simulink model "nivel_1"  (R2023b)
settings: Solver=FixedStepAuto  StartTime=0.0  StopTime=60  FixedStep=0.001  RelTol=1e-3
undefined symbols (not defined in the file): b_cx, b_cy, b_hb, b_hEb, b_hwu, b_t, b_tb, b_tw, bh_eq, bh_eq_prima, bt_eq, CI, ddx_t_lim, ddy_h_lim, DiscIntNeverNeededParam, dx_t_lim, dy_h_lim, g, H_c, H_SS, i_h, i_t, Jh_eq, Jh_eq_aux, Jt_eq, K_cy, K_hwu, K_tw, Kd_h, Kd_t, Ki_h, Ki_t, Kp_h, Kp_t, L_h0, M_cmax, M_s, m_t, r_hd, r_td, T_hb_max, T_hEb_max, T_hm_max, T_s1, T_s2, T_tb_max, T_tm_max, tau_hm, tau_tm, W_c, x_t_lim, Y_c, y_h_lim, Y_t0
libraries: simulink x19, dspstat3 x1, sldrtlib x1, simulink_extras x1
(part 2 of 2)

== stateflow chart nivel_1/Nivel 1 ==
  state Controlador
    entry:
    y_c = Y_c;
    state Mapeo_entradas_digitales [parallel]
      during:
      % Seleccion de operacion
      seleccion_oper = inputs(1);
      % Seleccion de muelle
      n_muelle = inputs(2);
      % Seleccion de posiciones en barco (+1 por sill beam)
      p_ini = inputs(3) + 1;
      p_fin = inputs(4) + 1;
      % Comandos del joystick
      joy_up = inputs(5);
      joy_down = inputs(6);
      % Modo de twistlocks (TLK)
      modo_tlk = inputs(7);
      % Inicio de operacion
      ini_oper = inputs(8);
      % Limit switches
      LLS_xt = limit_switches(1);
      RLS_xt = limit_switches(2);
      LELS_xt = limit_switches(3);
      RELS_xt = limit_switches(4);
      LLS_yt = limit_switches(5);
      RLS_yt = limit_switches(6);
      LELS_yt = limit_switches(7);
      RELS_yt = limit_switches(8);
      OS_izaje = limit_switches(15);
      settings: executionOrder=1
    state Operacion [parallel]
      settings: executionOrder=2
      note: Segun seleccion del operario
          | 0. Volver a home
          | Buscar carga en el muelle y llevar al barco
          | Buscar carga en barco y llevar al muelle
          | Mover carga dentro del barco
          | Reconocimiento de obstaculos
      state StandBy_home
        % Spreader en posicion de home
        % Espera hasta que el operador seleccione una operacion y la inicie
        % Siempre frenos puestos
        entry:
        BRK_h = false;
        BRK_t = false;
        fin_oper = false;
      state Reconocimiento_obstaculos
        % Se realiza recorrido desde x = 0 hasta limite (x = 50 - W_c/2) y se vuelve a posicion de SB (x = 0)
        entry:
        [x_t_vec, dx_t_vec] = perfil_velocidad_trapezoidal(T_s1, 0, 0, (x_t_lim(2) - W_c/2) ,0, set_param_lim(3), set_param_lim(4));
        BRK_t = true;
        flag_recon = 0;
        state Recorrido
          entry:
          idx_t = 1;
          during:
          % Paso de consigna de CARRO
          x_t = x_t_vec(idx_t);
          dx_t = dx_t_vec(idx_t);
          if idx_t  ~=  length(x_t_vec)
          idx_t = idx_t + 1;
          else
          flag_recon = flag_recon + 1;
          end
        state Vuelta
          entry:
          x_t_vec = flip(x_t_vec);
          dx_t_vec = -dx_t_vec;
          flag_recon = flag_recon + 1;
        (default) -> Recorrido
        Recorrido -> Vuelta : [flag_recon == 1]
        Vuelta -> Recorrido
      state Posicionamiento_desde_home
        % Se posiciona el spreader segun el tipo de accion partiendo desde home
        % Segun la seleccion del oeprador hay que posicionarse en muelle o barco
        % En funciones de homing, TIPO
        %     0 ->  IR A HOME
        %     1 -> SALIR DESDE HOME
        state StandBy
          entry:
          % Se abren frenos de izaje y carro
          BRK_h = true;
          BRK_t = true;
          flag = 0;
        state A_muelle
          entry:
          [carro_cons, izaje_cons, t_brk_t] = homing_muelle(T_s1, y_c_alt, W_c, H_c, set_param_lim, H_SS, tipo, n_muelle, -set_param_lim(3) * 0.5);
        state Salida_consignas
          entry:
          idx = 1;
          flag = 0;
          t_aux = clock;
          % =======================
          during:
          % Consignas de carro
          x_t = carro_cons(idx, 1);
          dx_t = carro_cons(idx, 2);
          % Consignas de izaje
          y_h = izaje_cons(idx, 1);
          dy_h = izaje_cons(idx, 2);
          if idx  ~=  length(izaje_cons)
          idx = idx + 1;
          end
          if idx == length(carro_cons)
          flag = 1;
          end
          % Freno de carro en caso de ser necesario
          if clock - t_aux > t_brk_t
          BRK_t = false;
          end
        state A_barco
          entry:
          [carro_cons, izaje_cons, t_brk_t] = homing_barco(T_s1, y_c_alt, W_c, set_param_lim, 1.5 * H_SS, tipo, p_ini, -1);
        (default) -> Controlador.Operacion.Posicionamiento_desde_home.StandBy
        Controlador.Operacion.Posicionamiento_desde_home.StandBy -> Controlador.Operacion.Posicionamiento_desde_home.A_muelle [order 2] : [seleccion_oper == 1]
        Controlador.Operacion.Posicionamiento_desde_home.A_muelle -> Controlador.Operacion.Posicionamiento_desde_home.Salida_consignas
        Controlador.Operacion.Posicionamiento_desde_home.StandBy -> Controlador.Operacion.Posicionamiento_desde_home.A_barco [order 1] : [seleccion_oper == 2]
        Controlador.Operacion.Posicionamiento_desde_home.A_barco -> Controlador.Operacion.Posicionamiento_desde_home.Salida_consignas
      state Posicionamiento_a_homing
        % Se posiciona el spreader segun el tipo de accion partiendo desde home
        % Segun la seleccion del oeprador hay que posicionarse en muelle o barco
        % En funciones de homing, TIPO
        %     0 ->  IR A HOME
        %     1 -> SALIR DESDE HOME
        tipo = 1;
        state StandBy
          entry:
          % Se abren frenos de izaje y carro
          BRK_h = true;
          BRK_t = true;
          flag = 0;
        state A_muelle
          entry:
          [carro_cons, izaje_cons, t_brk_t] = homing_muelle(T_s1, y_c_alt, W_c, H_c, set_param_lim, H_SS, tipo, n_muelle, -set_param_lim(3) * 0.5);
        state Salida_consignas
          entry:
          idx = 1;
          flag = 0;
          t_aux = clock;
          % =======================
          during:
          % Consignas de carro
          x_t = carro_cons(idx, 1);
          dx_t = carro_cons(idx, 2);
          % Consignas de izaje
          y_h = izaje_cons(idx, 1);
          dy_h = izaje_cons(idx, 2);
          if idx  ~=  length(izaje_cons)
          idx = idx + 1;
          end
          if idx == length(carro_cons)
          flag = 1;
          end
          % Freno de carro en caso de ser necesario
          if clock - t_aux > t_brk_t
          BRK_t = false;
          end
        state A_barco
          entry:
          [carro_cons, izaje_cons, t_brk_t] = homing_barco(T_s1, y_c_alt, W_c, set_param_lim, 1.5 * H_SS, tipo, p_ini, -1);
        (default) -> Controlador.Operacion.Posicionamiento_a_homing.StandBy
        Controlador.Operacion.Posicionamiento_a_homing.StandBy -> Controlador.Operacion.Posicionamiento_a_homing.A_muelle [order 2] : [seleccion_oper == 1]
        Controlador.Operacion.Posicionamiento_a_homing.A_muelle -> Controlador.Operacion.Posicionamiento_a_homing.Salida_consignas
        Controlador.Operacion.Posicionamiento_a_homing.StandBy -> Controlador.Operacion.Posicionamiento_a_homing.A_barco [order 1] : [seleccion_oper == 2]
        Controlador.Operacion.Posicionamiento_a_homing.A_barco -> Controlador.Operacion.Posicionamiento_a_homing.Salida_consignas
      note: Los pasos en las operaciones (una vez se realizo el posicionamiento) se enumeran como
          | Descenso manual
          | Cambio en modo de TLK (cierre)
          | Ascenso manual
          | Operacion automatica
          | Vuelta al paso 1
      state Modo_manual
        state Comprobacion_carga
          % Se realiza una comprobacion del peso del container al momento de realizar el izaje
          entry:
          t_aux = clock;
          state Levantamiento_carga
            % Se acelera hasta llegar a velocidad constante y se comprueba el peso
            during:
            if dy_h <= 0.5
            dy_h = (ddy_h_lim_man * T_s1) + dy_h;
            end
            y_h = p_izaje - H_c;
          state Descenso_por_sobrecarga
            % Se realiza descenso en velocidad reducida hasta F_hw = 0
            % y se activa alarma por sobrecarga
            during:
            if dy_h >= -0.5
            dy_h = -(ddy_h_lim * T_s1) + dy_h;
            end
            y_h = p_izaje - H_c;
            sobrecarga = true;
          state Calculo_carga
            % Calculo de tolerancia maxima de 5%
            entry:
            tol = M_cmax * 0.05;
            M_calc = (((2* F_hw) / g) - M_s);
          (default) -> Controlador.Operacion.Modo_manual.Comprobacion_carga.Levantamiento_carga
          Controlador.Operacion.Modo_manual.Comprobacion_carga.Levantamiento_carga -> Controlador.Operacion.Modo_manual.Comprobacion_carga.Calculo_carga : [clock - t_aux >= 3]
          Controlador.Operacion.Modo_manual.Comprobacion_carga.Calculo_carga -> Descenso_por_sobrecarga [order 1] : [M_calc >= M_cmax + tol]
        state StandBy
          % Se espera comando de subida o de bajada
          % Existen dos casos dentro del modo manual
          %    1 - Descenso desde altura segura, se limita seguridad
          %         Se realiza paro por inactividad del operario
          %         El descenso manual finaliza cuando F_hw == 0 (apoyo)
          %    2 - Ascenso hasta altura segura, se limita la velocidad de izaje
          % ==============
          entry:
          % Limites en la aceleracion y velocidad de izaje
          dy_h_lim_man = set_param_lim(3) * 0.5;
          ddy_h_lim_man = set_param_lim(4) * 0.5;
          y_h_aux = p_izaje;
        state Paro_inactividad
          % En caso de no tomar los controles se desacelera y se frena en v_0
          during:
          if dy_h <= 0
          dy_h = (ddy_h_lim_man * T_s1) + dy_h;
          else
          dy_h = 0;
          BRK_h = false;
          end
          y_h = p_izaje - (TLK * H_c);
        state Descenso_manual
          % Se realiza descenso progresivo hasta que se haga contacto con el container (F_hw == 0)
          % El descenso es a velocidad limitada, por cada que se mueve la palanca se genera una rampa de velocidad
          state Rampa_desc_velocidad
            during:
            dy_h = -(ddy_h_lim_man * T_s1) + dy_h;
            y_h = p_izaje - (TLK * H_c);
          state Rampa_asc_velocidad
            during:
            dy_h = (ddy_h_lim_man * T_s1) + dy_h;
            y_h = p_izaje - (TLK * H_c);
          state V_ctte
            during:
            y_h = p_izaje - (TLK * H_c);
            if dy_h >= 0
            dy_h = 0;
            elseif dy_h <= -dy_h_lim_man
            dy_h = -dy_h_lim_man;
            end
          (default) -> Controlador.Operacion.Modo_manual.Descenso_manual.Rampa_desc_velocidad
          Controlador.Operacion.Modo_manual.Descenso_manual.Rampa_desc_velocidad -> Controlador.Operacion.Modo_manual.Descenso_manual.Rampa_asc_velocidad [order 1] : [joy_down == 0]
          Controlador.Operacion.Modo_manual.Descenso_manual.Rampa_asc_velocidad -> Controlador.Operacion.Modo_manual.Descenso_manual.Rampa_desc_velocidad [order 2] : [joy_down == 1 && dy_h > -dy_h_lim_man]
          Controlador.Operacion.Modo_manual.Descenso_manual.V_ctte -> Controlador.Operacion.Modo_manual.Descenso_manual.Rampa_desc_velocidad [order 2] : [joy_down == 1 && dy_h < -dy_h_lim_man]
          Controlador.Operacion.Modo_manual.Descenso_manual.Rampa_desc_velocidad -> Controlador.Operacion.Modo_manual.Descenso_manual.V_ctte [order 2] : [dy_h <= -dy_h_lim_man]
          Controlador.Operacion.Modo_manual.Descenso_manual.Rampa_asc_velocidad -> Controlador.Operacion.Modo_manual.Descenso_manual.V_ctte [order 1] : [dy_h >= 0]
          Controlador.Operacion.Modo_manual.Descenso_manual.V_ctte -> Controlador.Operacion.Modo_manual.Descenso_manual.Rampa_asc_velocidad [order 1] : [joy_down == 0 && dy_h ~= 0]
        state Ascenso_manual
          % Se realiza descenso progresivo hasta que se haya contacto con el container (F_hw == 0)
          % El descenso es a velocidad limitada, por cada que se mueve la palanca se genera una rampa de velocidad
          paso = 3;
          state Rampa_asc_velocidad
            during:
            dy_h = (ddy_h_lim_man * T_s1) + dy_h;
            y_h = p_izaje - (TLK * H_c);
          state Rampa_desc_velocidad
            during:
            dy_h = -(ddy_h_lim_man * T_s1) + dy_h;
            y_h = p_izaje - (TLK * H_c);
          state V_ctte
            during:
            y_h = p_izaje - (TLK * H_c);
            if dy_h <= 0
            dy_h = 0;
            elseif dy_h >= dy_h_lim_man
            dy_h = dy_h_lim_man;
            end
          (default) -> Controlador.Operacion.Modo_manual.Ascenso_manual.Rampa_asc_velocidad
          Controlador.Operacion.Modo_manual.Ascenso_manual.Rampa_asc_velocidad -> Controlador.Operacion.Modo_manual.Ascenso_manual.Rampa_desc_velocidad [order 2] : [joy_up == 0]
          Controlador.Operacion.Modo_manual.Ascenso_manual.Rampa_desc_velocidad -> Controlador.Operacion.Modo_manual.Ascenso_manual.Rampa_asc_velocidad [order 2] : [joy_up == 1 && dy_h < dy_h_lim_man]
          Controlador.Operacion.Modo_manual.Ascenso_manual.V_ctte -> Controlador.Operacion.Modo_manual.Ascenso_manual.Rampa_asc_velocidad [order 2] : [joy_up == 1 && dy_h < dy_h_lim_man]
          Controlador.Operacion.Modo_manual.Ascenso_manual.Rampa_asc_velocidad -> Controlador.Operacion.Modo_manual.Ascenso_manual.V_ctte [order 1] : [dy_h >= dy_h_lim_man]
          Controlador.Operacion.Modo_manual.Ascenso_manual.Rampa_desc_velocidad -> Controlador.Operacion.Modo_manual.Ascenso_manual.V_ctte [order 1] : [dy_h <= 0]
          Controlador.Operacion.Modo_manual.Ascenso_manual.V_ctte -> Controlador.Operacion.Modo_manual.Ascenso_manual.Rampa_desc_velocidad [order 1] : [joy_up == 0 && dy_h ~= 0]
        (default) -> Controlador.Operacion.Modo_manual.StandBy
        (junction 383) -> Controlador.Operacion.Modo_manual.Comprobacion_carga [order 1] : [TLK == true]
        Controlador.Operacion.Modo_manual.StandBy -> (junction 383) [order 1] : [joy_up == 1 && paso == 2]
            | {BRK_h = true,
            | paso = 3;}
        (junction 383) -> Controlador.Operacion.Modo_manual.Ascenso_manual [order 2] : [TLK == false ]
        Controlador.Operacion.Modo_manual.Comprobacion_carga.Calculo_carga -> Controlador.Operacion.Modo_manual.Ascenso_manual [order 2] : [M_calc < M_cmax + tol]
        Controlador.Operacion.Modo_manual.StandBy -> (junction 327) [order 2] : [paso == 1]
        (junction 327) -> Controlador.Operacion.Modo_manual.Paro_inactividad [order 1] : [joy_down == 0]
        (junction 327) -> Controlador.Operacion.Modo_manual.Descenso_manual [order 2] : [joy_down == 1]
        Controlador.Operacion.Modo_manual.Paro_inactividad -> Controlador.Operacion.Modo_manual.Descenso_manual : [joy_down == 1]
            | {BRK_h = true;}
      state StandBy_posicionado
        % Spreader en posicion fuera de home (muelle o barco)
        % Espera hasta que el operador seleccione una operacion y la inicie
        % Siempre frenos puestos
        entry:
        BRK_h = false;
        BRK_t = false;
        fin_oper = false;
      state Apoyo
        % Dependiendo de los TLK
        %    TLK = true -> container apoyado
        %    TLK = false -> spreader apoyado
        % Se aplica freno de izaje y se espera a comando del operador
        entry:
        fin_modo_TLK = false;
        y_h = p_izaje - (TLK * H_c);
        dy_h = 0;
        paso = 2;
        state Cierre_TLK
          % Se pretende tomar una carga
          % Se simula el cierre con 3 segundos de delay
          entry:
          t_aux = clock;
          exit:
          TLK = true;
          if seleccion_oper == 2
          y_c(pos_x) = y_c(pos_x) - 1;
          end
        state StandBy
          % A la espera del comando del operador
        state Fin_modo_TLK
          fin_modo_TLK = true;
        state Apertura_TLK
          % Se pretende soltar la carga
          % Se simula la apertura con 3 segundos de delay
          entry:
          t_aux = clock;
          exit:
          TLK = false;
          y_c(p_ini) = y_c(p_ini) + 1;
          fin_oper = true;
          if seleccion_oper == 1
          y_c(pos_x) = y_c(pos_x) + 1;
          end
        Controlador.Operacion.Apoyo.StandBy -> Controlador.Operacion.Apoyo.Cierre_TLK [order 2] : [TLK == false && modo_tlk == 1]
        (default) -> Controlador.Operacion.Apoyo.StandBy
        Controlador.Operacion.Apoyo.Cierre_TLK -> Controlador.Operacion.Apoyo.Fin_modo_TLK : [(clock - t_aux) >= 3 ]
        Controlador.Operacion.Apoyo.StandBy -> Controlador.Operacion.Apoyo.Apertura_TLK [order 1] : [TLK == true && modo_tlk == 0]
        Controlador.Operacion.Apoyo.Apertura_TLK -> Controlador.Operacion.Apoyo.Fin_modo_TLK : [(clock - t_aux) >= 3]
      state Modo_automatico
        % Dependiendo del tipo de operacion (seleccion_oper) se cambia el valor del tipo
        %     tipo = 0 -> Descarga desde barco al muelle
        %     tipo = 1 -> Carga desde muelle a barco
        %     tipo = 2 -> Movimiento dentro del barco
        % Luego se utiliza la variable paso para determinar si es posicionamiento o toma de carga/descarga
        state Salida_consignas
          entry:
          idx = 1;
          flag = 0;
          t_aux = clock;
          % =======================
          during:
          % Consignas de carro
          x_t = carro_cons(idx, 1);
          dx_t = carro_cons(idx, 2);
          % Consignas de izaje
          y_h = izaje_cons(idx, 1);
          dy_h = izaje_cons(idx, 2);
          if idx  ~=  length(izaje_cons)
          idx = idx + 1;
          end
          if idx == length(carro_cons)
          flag = 1;
          end
          % Freno de carro en caso de ser necesario
          if clock - t_aux > t_brk_t
          BRK_t = false;
          end
        state Condicionantes
          entry:
          if seleccion_oper == 0
          % Descarga desde barco a muelle
          tipo = 0;
          elseif seleccion_oper == 1
          % Carga desde muelle a barco
          tipo = 1;
          else
          % Operacion intra-barco
          tipo = 2;
          end
        state Consignas_automatico
          entry:
          [carro_cons, izaje_cons, t_brk_t, t_brk_h] = operacion_automatico(T_s1, y_c_alt, W_c, H_c, TLK, set_param_lim, H_SS, tipo, n_muelle, p_ini, p_fin, dy_h, set_param_lim(3));
        (default) -> Controlador.Operacion.Modo_automatico.Condicionantes
        Controlador.Operacion.Modo_automatico.Condicionantes -> Consignas_automatico
        Consignas_automatico -> Controlador.Operacion.Modo_automatico.Salida_consignas
      state Posicionamiento_automatico
        % El spreader esta fuera de homing, pero o esta dentro del barco o en muelle
        % Entonces dependiende de la seleccion del operador, y las condiciones de posicionamiento del spreader, se usa una de las siguientes funciones
        %
        % Spreader esta en barco y operador selecciona operacion de muelle a barco (o viceversa, spreader en muelle y operacion barco a muelle)
        %   operacion_automatico (tipo 0 y 1)
        %
        % Spreader esta en barco y operador selecciona de barco a muelle
        %   operacion_automatico (tipo 2)
        %
        % Spreader esta en muelle y operador selecciona de muelle a barco
        %   cambia_muelle
        entry:
        BRK_t = true;
        BRK_h = true;
        state Salida_consignas
          entry:
          idx = 1;
          flag = 0;
          t_aux = clock;
          % =======================
          during:
          % Consignas de carro
          x_t = carro_cons(idx, 1);
          dx_t = carro_cons(idx, 2);
          % Consignas de izaje
          y_h = izaje_cons(idx, 1);
          dy_h = izaje_cons(idx, 2);
          if idx  ~=  length(izaje_cons)
          idx = idx + 1;
          end
          if idx == length(carro_cons)
          flag = 1;
          end
          % Freno de carro en caso de ser necesario
          if clock - t_aux > t_brk_t
          BRK_t = false;
          end
        state Condicionantes
          entry:
          tipo = -1;
          if x_t < 0 && seleccion_oper == 2 || seleccion_oper == 3
          tipo = 1;
          elseif x_t > 0 && seleccion_oper == 1
          tipo = 0;
          elseif x_t > 0 && seleccion_oper == 3
          tipo = 2;
          end
        state Posicionamiento_en_muelle
          entry:
          % Calculo del muelle actual
          n_muelle_act = fix(abs(p_carro) / (2 * W_c)) + 1;
          [carro_cons, izaje_cons, t_brk_t, t_brk_h] = cambio_muelle(T_s1, W_c, H_c, set_param_lim, H_SS, n_muelle_act, n_muelle, 0)
        state Posicionamiento_combinado
          entry:
          [carro_cons, izaje_cons, t_brk_t, t_brk_h] = operacion_automatico(T_s1, y_c_alt, W_c, H_c, TLK, set_param_lim, H_SS, tipo, n_muelle, p_ini, p_fin, dy_h, set_param_lim(3));
        Posicionamiento_en_muelle -> Controlador.Operacion.Posicionamiento_automatico.Salida_consignas
        (default) -> Controlador.Operacion.Posicionamiento_automatico.Condicionantes
        Controlador.Operacion.Posicionamiento_automatico.Condicionantes -> Posicionamiento_en_muelle [order 1] : [tipo == -1]
        Posicionamiento_combinado -> Controlador.Operacion.Posicionamiento_automatico.Salida_consignas
        Controlador.Operacion.Posicionamiento_automatico.Condicionantes -> Posicionamiento_combinado [order 2] : [tipo ~= -1]
      (default) -> StandBy_home
      StandBy_home -> Reconocimiento_obstaculos [order 2] : [seleccion_oper == 4 && ini_oper == 1]
      Posicionamiento_a_homing -> StandBy_home : [flag == 1]
      Reconocimiento_obstaculos -> StandBy_home : [flag_recon == 3]
          | {flag_recon = 0;}
      StandBy_home -> Posicionamiento_desde_home [order 1] : [(seleccion_oper >= 1 && seleccion_oper <= 3) && ini_oper == 1]
      StandBy_posicionado -> Posicionamiento_a_homing [order 1] : [seleccion_oper == 0 && ini_oper == 1]
      Posicionamiento_desde_home -> Controlador.Operacion.Modo_manual : [flag == 1]
          | {paso = 1;}
      Controlador.Operacion.Modo_manual -> Apoyo [order 1] : [F_hw == 0]
          | {BRK_h = false;}
      Controlador.Operacion.Modo_manual -> StandBy_posicionado [order 3] : [((y_h_aux + H_SS) <= (y_h + (TLK * H_c))) && fin_oper == true]
      Apoyo -> Controlador.Operacion.Modo_manual : [fin_modo_TLK == true]
      Posicionamiento_automatico -> Controlador.Operacion.Modo_manual : [flag == 1]
          | {paso = 1;}
      StandBy_posicionado -> Posicionamiento_automatico [order 2] : [(seleccion_oper >= 1 && seleccion_oper <= 3) && ini_oper == 1]
      Controlador.Operacion.Modo_automatico -> Controlador.Operacion.Modo_manual : [flag == 1]
          | {paso = 1;}
      Controlador.Operacion.Modo_manual -> Controlador.Operacion.Modo_automatico [order 2] : [paso == 3 && ((y_h_aux + H_SS) <= (y_h + (TLK * H_c))) ]
          | {BRK_t = true;
          | paso = 4;}
    state Mapeo_entradas_analogicas [parallel]
      during:
      % Sensores en motores
      p_carro = sensores(1);
      v_carro = sensores(2);
      p_izaje = sensores(3);
      v_izaje = sensores(4);
      settings: executionOrder=3
    state Mapeo_salidas_analogicas [parallel]
      during:
      % Calculo de y_c0 -------------------------
      pos_x = fix(abs(x_t / (2 * W_c))) + 1;
      % Encima de barco
      if x_t > 0 && pos_x <= length(y_c)
      y_c0 = y_c_alt(pos_x);
      % Fuera del barco
      elseif x_t < 0
      y_c0 = H_c * (~TLK);
      end
      % Calculo del peso de la carga
      M_calc_aux = ((2* F_hw) / g) - M_s;
      if M_calc_aux > M_cmax
      M_calc_aux = M_cmax;
      end
      settings: executionOrder=4
    state Auxiliares [parallel]
      during:
      % Segun modo de twistlocks se calculan limites de velocidad de izaje
      if TLK == true
      h_c = H_c;
      % Interpolacion para velocidad maxima segun la carga
      v_lim_carga = dy_h_lim(1) + (dy_h_lim(2) - dy_h_lim(1)) * (M_calc_aux / M_cmax);
      set_param_lim = [dx_t_lim ddx_t_lim v_lim_carga ddy_h_lim];
      else
      h_c = 0;
      set_param_lim = [dx_t_lim ddx_t_lim dy_h_lim(2) ddy_h_lim];
      end
      % Perfil de obstaculos en [m]
      y_c_alt = y_c * H_c;
      settings: executionOrder=5
  state Modo_manual [commented out]
    % En este estado se comanda la logica en modo manual, solo en casos de carga y descarga de containers
    state StandBy [commented out]
      % Existen tres casos dentro del modo manual
      %    1 - Descenso (v_h < 0)
      %    2 - Ascenso (cuando se carga/descarga)
      %    3 - Toma de carga (manejo de TLK)
    state Paro_inactividad [commented out]
      % En caso de no tomar los controles se aplican frenos y se espera comando del operador
      during:
      if dy_h < 0
      dy_h = (ddy_h_lim * T_s1) + dy_h;
      else
      dy_h = 0;
      BRK_h = false;
      end
      y_h = p_izaje;
    state Descenso_manual [commented out]
      % Se realiza descenso progresivo hasta que se haya contacto con el container (F_hw == 0)
      % El descenso es a velocidad limitada, por cada que se mueve la palanca se genera una rampa de velocidad
      entry:
      v_limite = -dy_h_lim(1);
      state Rampa_asc_velocidad [commented out]
        during:
        dy_h = -(ddy_h_lim * T_s1) + dy_h;
        y_h = p_izaje - (TLK * H_c);
      state Rampa_desc_velocidad [commented out]
        during:
        dy_h = (ddy_h_lim * T_s1) + dy_h;
        y_h = p_izaje - (TLK * H_c);
      state V_ctte [commented out]
        during:
        y_h = p_izaje - (TLK * H_c);
        if dy_h >= 0
        dy_h = 0;
        elseif dy_h <= v_limite
        dy_h = v_limite;
        end
      (default) -> Modo_manual.Descenso_manual.Rampa_asc_velocidad [commented out]
      Modo_manual.Descenso_manual.Rampa_asc_velocidad -> Modo_manual.Descenso_manual.Rampa_desc_velocidad [commented out] : [joy_down == 0]
      Modo_manual.Descenso_manual.Rampa_desc_velocidad -> Modo_manual.Descenso_manual.Rampa_asc_velocidad [commented out] : [joy_down == 1 && dy_h > v_limite]
      Modo_manual.Descenso_manual.V_ctte -> Modo_manual.Descenso_manual.Rampa_asc_velocidad [commented out] : [joy_down == 1 && dy_h > v_limite]
      Modo_manual.Descenso_manual.Rampa_asc_velocidad -> Modo_manual.Descenso_manual.V_ctte [commented out] : [dy_h <= v_limite]
      Modo_manual.Descenso_manual.V_ctte -> Modo_manual.Descenso_manual.Rampa_desc_velocidad [commented out] : [joy_down == 0 && dy_h ~= 0]
      Modo_manual.Descenso_manual.Rampa_desc_velocidad -> Modo_manual.Descenso_manual.V_ctte [commented out] : [dy_h >= 0]
    state Ascenso_manual [commented out]
      % Se realiza descenso progresivo hasta que se haya contacto con el container (F_hw == 0)
      % El descenso es a velocidad limitada, por cada que se mueve la palanca se genera una rampa de velocidad
      entry:
      v_limite = set_param_lim(3);
      state Rampa_asc_velocidad [commented out]
        during:
        dy_h = ddy_h_lim * T_s1 + dy_h;
        y_h = p_izaje - (TLK * H_c);
      state Rampa_desc_velocidad [commented out]
        during:
        dy_h = -(ddy_h_lim * T_s1) + dy_h;
        y_h = p_izaje - (TLK * H_c);
      state V_ctte [commented out]
        during:
        y_h = p_izaje - (TLK * H_c);
        if dy_h <= 0
        dy_h = 0;
        elseif dy_h >= v_limite
        dy_h = v_limite;
        end
      (default) -> Modo_manual.Ascenso_manual.Rampa_asc_velocidad [commented out]
      Modo_manual.Ascenso_manual.Rampa_asc_velocidad -> Modo_manual.Ascenso_manual.Rampa_desc_velocidad [commented out] : [joy_up == 0]
      Modo_manual.Ascenso_manual.Rampa_desc_velocidad -> Modo_manual.Ascenso_manual.Rampa_asc_velocidad [commented out] : [joy_up == 1 && dy_h < v_limite]
      Modo_manual.Ascenso_manual.V_ctte -> Modo_manual.Ascenso_manual.Rampa_asc_velocidad [commented out] : [joy_up == 1 && dy_h < v_limite]
      Modo_manual.Ascenso_manual.Rampa_asc_velocidad -> Modo_manual.Ascenso_manual.V_ctte [commented out] : [dy_h >= v_limite]
      Modo_manual.Ascenso_manual.V_ctte -> Modo_manual.Ascenso_manual.Rampa_desc_velocidad [commented out] : [joy_up == 0 && dy_h ~= 0]
      Modo_manual.Ascenso_manual.Rampa_desc_velocidad -> Modo_manual.Ascenso_manual.V_ctte [commented out] : [dy_h <= 0]
    state Apoyo_en_container [commented out]
      % Spreader apoyado en container, se procede a poner freno en izaje y enviar consigna de velocidad 0
      entry:
      BRK_h = false;
      y_h = p_izaje;
      dy_h = 0;
      state Cierre_TLK [commented out]
        % Se pretende tomar una carga
        % Se simula el cierre con 3 segundos de delay
        entry:
        t_aux = clock;
        exit:
        TLK = true;
      state StandBy [commented out]
        % A la espera en el
        % cambio en
        % modo_tlk
      state Fin_modo_TLK [commented out]
      state Apertura_TLK [commented out]
        % Se pretende soltar la carga
        % Se simula la apertura con 3 segundos de delay
        entry:
        t_aux = clock;
        exit:
        TLK = false;
      (default) -> Modo_manual.Apoyo_en_container.StandBy [commented out]
      Modo_manual.Apoyo_en_container.StandBy -> Modo_manual.Apoyo_en_container.Cierre_TLK [commented out] : [TLK == false && modo_tlk == 1]
      Modo_manual.Apoyo_en_container.Cierre_TLK -> Modo_manual.Apoyo_en_container.Fin_modo_TLK [commented out] : [(clock - t_aux) >= 3 ]
      Modo_manual.Apoyo_en_container.StandBy -> Modo_manual.Apoyo_en_container.Apertura_TLK [commented out] : [TLK == true && modo_tlk == 0]
      Modo_manual.Apoyo_en_container.Apertura_TLK -> Modo_manual.Apoyo_en_container.Fin_modo_TLK [commented out] : [(clock - t_aux) >= 3]
    state Comprobacion_carga [commented out]
      % Se realiza una comprobacion del peso del container al momento de realizar el izaje
      entry:
      t_aux = clock;
      state Levantamiento_carga [commented out]
        % Se acelera hasta llegar a velocidad constante y se comprueba el peso
        during:
        if dy_h <= 0.5
        dy_h = (ddy_h_lim * T_s1) + dy_h;
        end
        y_h = p_izaje - H_c;
      state Calculo_carga [commented out]
        % Calculo de tolerancia maxima de 5%
        entry:
        tol = 5 / 100;
        M_calc = (((2* F_hw) / g) - M_s);
      state Descenso_por_sobrepeso [commented out]
        % Se realiza descenso hasta F_hw = 0
        during:
        if dy_h >= -0.5
        dy_h = -(ddy_h_lim * T_s1) + dy_h;
        end
        y_h = p_izaje - H_c;
      Modo_manual.Comprobacion_carga.Levantamiento_carga -> Modo_manual.Comprobacion_carga.Calculo_carga [commented out] : [clock - t_aux >= 3]
      (default) -> Modo_manual.Comprobacion_carga.Levantamiento_carga [commented out]
      Modo_manual.Comprobacion_carga.Calculo_carga -> Descenso_por_sobrepeso [commented out] : [M_calc > M_cmax + (M_cmax * (1 + tol))]
    state Apertura_automatica_TLK_por_sobrepeso [commented out]
      entry:
      TLK = false;
      y_h = p_izaje;
      t_aux = clock;
    (default) -> Modo_manual.StandBy [commented out]
    Modo_manual.StandBy -> (junction 145) [commented out] : [dy_h < 0]
    (junction 145) -> Modo_manual.Paro_inactividad [commented out] : [joy_down == 0]
    (junction 145) -> Modo_manual.Descenso_manual [commented out] : [joy_down == 1]
    Modo_manual.Paro_inactividad -> Modo_manual.Descenso_manual [commented out] : [joy_down == 1]
        | {BRK_h = true;}
    Modo_manual.Descenso_manual -> Apoyo_en_container [commented out] : [F_hw == 0]
    Modo_manual.Apoyo_en_container.Fin_modo_TLK -> Modo_manual.Ascenso_manual [commented out] : [TLK == false && joy_up == 1]
        | {BRK_h = true;}
    Modo_manual.Comprobacion_carga.Calculo_carga -> Modo_manual.Ascenso_manual [commented out] : [M_calc <= (M_cmax * (1 + tol)) && joy_up == 1]
    Modo_manual.Apoyo_en_container.Fin_modo_TLK -> Modo_manual.Comprobacion_carga [commented out] : [TLK == true && joy_up == 1]
        | {BRK_h = true;}
    Descenso_por_sobrepeso -> Apertura_automatica_TLK_por_sobrepeso [commented out] : [F_hw == 0]
  state Modo_automatico [commented out]
    state Accion_carga_automatico [commented out]
      state Calculos_auxiliares [commented out]
        % Calculos para realizar las maniobras pertinentes
        y_max = (max(y_c(1:p_fin)) * H_c) + H_SS;
      state Toma_carga_muelle_automatico [commented out]
        % Se toma carga desde posicion en muelle y se lleva al barco
        % -------------
        entry:
        [carro_cons, izaje_cons] = consigna_en_muelle(T_s1, W_c, set_param_lim, n_muelle, y_max , H_SS, 0, dy_h, 1);
        idx_t = 1; idx_h = 1;
        flag = 0;
        % -------------
        during:
        % Carro
        x_t = carro_cons(idx_t, 1);
        dx_t = carro_cons(idx_t, 2);
        % Izaje
        y_h = izaje_cons(idx_h, 1);
        dy_h = izaje_cons(idx_h, 2);
        if idx_t  ~=  length(carro_cons)
        idx_t = idx_t + 1;
        end
        if idx_h  ~=  length(izaje_cons)
        idx_h = idx_h + 1;
        end
        if idx_t == length(carro_cons) && idx_h == length(izaje_cons)
        flag = 1;
        end
      state Deja_carga_barco [commented out]
        % Se entra con v_t y deja carga en barco
        % -------------
        entry:
        [carro_cons, izaje_cons] = consigna_en_barco(T_s1, W_c, H_c, y_c, set_param_lim, p_ini, 0, H_SS, dx_t, 0, 1);
        idx_t = 1; idx_h = 1;
        flag = 0;
        % -------------
        during:
        % Carro
        x_t = carro_cons(idx_t, 1);
        dx_t = carro_cons(idx_t, 2);
        % Izaje
        y_h = izaje_cons(idx_h, 1) - (TLK * H_c);
        dy_h = izaje_cons(idx_h, 2);
        if idx_t  ~=  length(carro_cons)
        idx_t = idx_t + 1;
        end
        if idx_h  ~=  length(izaje_cons)
        idx_h = idx_h + 1;
        end
        if idx_t == length(carro_cons) && idx_h == length(izaje_cons)
        flag = 2;
        end
      (default) -> Modo_automatico.Accion_carga_automatico.Calculos_auxiliares [commented out]
      Modo_automatico.Accion_carga_automatico.Calculos_auxiliares -> Toma_carga_muelle_automatico [commented out]
      Toma_carga_muelle_automatico -> Deja_carga_barco [commented out] : [flag == 1]
    state Accion_descarga_automatico [commented out]
      state Calculos_auxiliares [commented out]
        % Calculos para realizar las maniobras pertinentes
        y_max = (max(y_c(1:p_fin)) * H_c) + H_SS;
      state Toma_carga_barco [commented out]
        % Sale del barco a v_t y se dirije hacia muelle con carga
        % -------------
        entry:
        [carro_cons, izaje_cons] = consigna_en_barco(T_s1, W_c, H_c, y_c, set_param_lim, p_ini, 0, H_SS, dx_t, dy_h, 0);
        idx_t = 1; idx_h = 1;
        flag = 0;
        % -------------
        during:
        % Carro
        x_t = carro_cons(idx_t, 1);
        dx_t = carro_cons(idx_t, 2);
        % Izaje
        y_h = izaje_cons(idx_h, 1);
        dy_h = izaje_cons(idx_h, 2);
        if idx_t  ~=  length(carro_cons)
        idx_t = idx_t + 1;
        end
        if idx_h  ~=  length(izaje_cons)
        idx_h = idx_h + 1;
        end
        if idx_t == length(carro_cons) && idx_h == length(izaje_cons)
        flag = 2;
        end
      state Deja_carga_muelle_automatico [commented out]
        % Se toma carga desde posicion en muelle y se lleva al barco
        % -------------
        entry:
        [carro_cons, izaje_cons] = consigna_en_muelle(T_s1, W_c, set_param_lim, n_muelle, y_max , H_SS, dx_t, dy_h, 0);
        idx_t = 1; idx_h = 1;
        flag = 0;
        % -------------
        during:
        % Carro
        x_t = carro_cons(idx_t, 1);
        dx_t = carro_cons(idx_t, 2);
        % Izaje
        y_h = izaje_cons(idx_h, 1);
        dy_h = izaje_cons(idx_h, 2);
        if idx_t  ~=  length(carro_cons)
        idx_t = idx_t + 1;
        end
        if idx_h  ~=  length(izaje_cons)
        idx_h = idx_h + 1;
        end
        if idx_t == length(carro_cons) && idx_h == length(izaje_cons)
        flag = 1;
        end
      (default) -> Modo_automatico.Accion_descarga_automatico.Calculos_auxiliares [commented out]
      Modo_automatico.Accion_descarga_automatico.Calculos_auxiliares -> Toma_carga_barco [commented out]
      Toma_carga_barco -> Deja_carga_muelle_automatico [commented out] : [flag == 1]
    state Homing [commented out]
  (default) -> Controlador
  Accion_carga_automatico -> Modo_manual.Descenso_manual [commented out] : [flag == 2]
  Modo_manual.Ascenso_manual -> Accion_carga_automatico [commented out] : [seleccion_oper == 1 && y_h >= H_SS ]
      | {BRK_t = true;}
  Modo_manual.Ascenso_manual -> Accion_descarga_automatico [commented out] : [seleccion_oper == 2 && dy_h > H_SS]
  data: sensores input; limit_switches input; inputs input size=8; F_hw input; T_s1 parameter; carro_cons local size=[10000; 10000] =[CI(1) CI(2)]; izaje_cons local size=[10000; 10000] =[CI(3) CI(4)]; W_c parameter; ddx_t_lim parameter; ddy_h_lim parameter; dx_t_lim parameter; dy_h_lim parameter; H_SS parameter; v_act local; set_param_lim local; n_muelle local; altura_izaje local; flag local =0; idx_h local =1; idx_t local =1; dx_t output size=1 =CI(2); dy_h output size=1 =CI(4); x_t output size=1 =CI(1); y_h output size=1 =CI(3); clock input; H_c parameter; p_ini local; p_fin local; y_c local; y_max local; CI parameter; seleccion_oper local; BRK_t output boolean =false; BRK_h output boolean =false; BRK_hE output boolean =true; calc_aux local; t_aux local; joy_down local; joy_up local; dy_h_vec local size=[10000; 10000]; y_h_vec local size=[10000; 10000]; TLK output boolean =false; y_c0 output =0; OS_izaje local; RLS_yt local; RLS_xt local; RELS_yt local; RELS_xt local; LLS_yt local; LLS_xt local; LELS_yt local; LELS_xt local; p_carro local; p_izaje local; v_carro local; v_izaje local; v_limite local; T_s2 parameter; x_t_lim parameter; dx_t_vec local size=[10000; 10000]; flag_recon local =0; x_t_vec local size=[10000; 10000]; pos_x local; y_obj local; h_c local; modo_tlk local; dy_h_lim_aux local =dy_h_lim(2); Y_c parameter; M_s parameter; g parameter; M_calc output; ini_oper local =0; M_cmax parameter; v_lim_carga local; tol local; M_calc_aux local; tipo local; idx local; t_brk_t local; ddy_h_lim_man local; dy_h_lim_man local; fin_modo_TLK local =false; paso local; y_h_aux local; y_c_alt local; t_brk_h local; sobrecarga local; fin_oper local
